simulink model "metoda2_bezposrednia"  (R2017b)
settings: Solver=VariableStepAuto  StartTime=0.0  StopTime=10.0  RelTol=1e-3
values from neighbouring files (symbols this model uses):
  A2 = A1'    [initial_values.m]    (also in matlab.mat = [3.22791678547  1  0; -1.44925930399  0  1; 0.17377394345  0)
  B2 = C1'    [initial_values.m]    (also in matlab.mat = [0.260707487539 -0.289205764977 0.0761198486843])
  Tp = 0.25    [initial_values.m]    (also in matlab.mat)
settings Model: Creator=Paweł  LastModifiedBy=Paweł

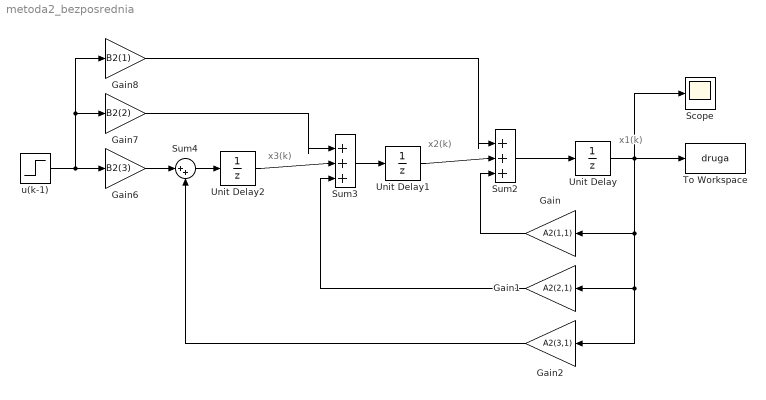
== system metoda2_bezposrednia ==
  note: x1(k)
  note: x2(k)
  note: x3(k)
  Gain : Gain  Gain=A2(1,1)
  Gain1 : Gain  Gain=A2(2,1)
  Gain2 : Gain  Gain=A2(3,1)
  Gain6 : Gain  Gain=B2(3)
  Gain7 : Gain  Gain=B2(2)
  Gain8 : Gain  Gain=B2(1)
  Scope : Scope
  Sum2 : Sum  Inputs=|+++
  Sum3 : Sum  Inputs=|+++
  Sum4 : Sum  Inputs=|++
  To Workspace : ToWorkspace  VariableName=druga  SaveFormat=Timeseries  SampleTime=-1
  Unit Delay : UnitDelay  SampleTime=Tp
  Unit Delay1 : UnitDelay  SampleTime=Tp
  Unit Delay2 : UnitDelay  SampleTime=Tp
  u(k-1) : Step  SampleTime=0
  wires:
  Gain6/1 -> Sum4/1
  Unit Delay2/1 -> Sum3/2
  Gain2/1 -> Sum4/2
  Gain/1 -> Sum2/3
  Gain8/1 -> Sum2/1
  Sum4/1 -> Unit Delay2/1
  Gain1/1 -> Sum3/3
  Gain7/1 -> Sum3/1
  Sum3/1 -> Unit Delay1/1
  Unit Delay1/1 -> Sum2/2
  Unit Delay/1 -> Scope/1, To Workspace/1, Gain2/1, Gain1/1, Gain/1
  Sum2/1 -> Unit Delay/1
  u(k-1)/1 -> Gain8/1, Gain7/1, Gain6/1
